simulink model "MATLAB_Function"  (R2022a)
settings: Solver=FixedStepAuto  StartTime=0.0  StopTime=10.0  FixedStep=1/1e4  RelTol=1e-3
settings Model: Creator=basti  LastModifiedBy=milan
settings DataIOCC: SaveOutput=off  SaveTime=off
settings DebuggingCC: UnconnectedInputMsg=warning  UnconnectedOutputMsg=warning  UnconnectedLineMsg=warning
settings RTWCC: DLArmComputeVersion=19.05

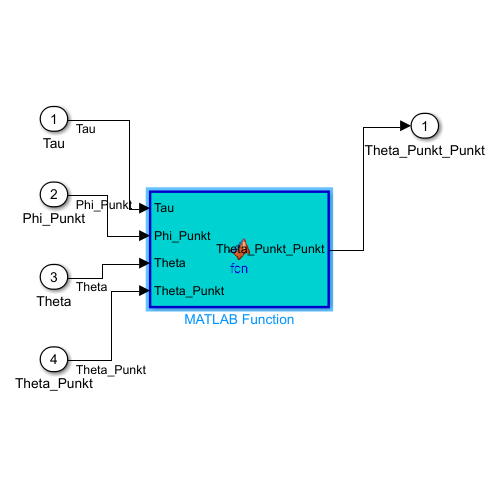
[thumbnail: Simulink's stored preview of the top-level diagram]
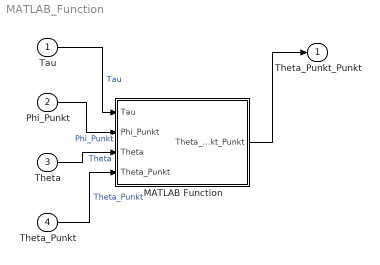
== system MATLAB_Function ==
  Tau : Inport  OutDataTypeStr=double  PortDimensions=1  SampleTime=0
  Phi_Punkt : Inport  Port=2  OutDataTypeStr=double  PortDimensions=1  SampleTime=0
  Theta : Inport  Port=3  OutDataTypeStr=double  PortDimensions=1  SampleTime=0
  Theta_Punkt : Inport  Port=4  OutDataTypeStr=double  PortDimensions=1  SampleTime=0
  MATLAB Function : MATLAB Function  TreatAsAtomicUnit=on
  Theta_Punkt_Punkt : Outport  OutDataTypeStr=double  PortDimensions=1  SampleTime=0
  wires:
  Tau/1 -> MATLAB Function/1(Tau)  "Tau"
  Phi_Punkt/1 -> MATLAB Function/2(Phi_Punkt)  "Phi_Punkt"
  Theta/1 -> MATLAB Function/3(Theta)  "Theta"
  Theta_Punkt/1 -> MATLAB Function/4(Theta_Punkt)  "Theta_Punkt"
  MATLAB Function/1(Theta_Punkt_Punkt) -> Theta_Punkt_Punkt/1

== matlab function MATLAB_Function/MATLAB Function ==
  data: Tau input; Theta_Punkt_Punkt output; Phi_Punkt input; Theta input; Theta_Punkt input; c parameter
function Theta_Punkt_Punkt = fcn(Tau, Phi_Punkt, Theta, Theta_Punkt,c)
    % Konstanten aufrufen
    %c = Konstanten();
    
    % Berechnung
    Theta_Punkt_Punkt = ((Tau-c.c2*Phi_Punkt-(c.m1*c.l1+c.m2*c.l2)*c.g*sin(Theta)+c.c1*Theta_Punkt)/c.J2)/(1-(c.m1*c.l1^2+c.m2*c.l2^2+c.J1+c.J2)/c.J2);
